simulink model "Mechanical_part_only"  (Simulink 7.5)
settings: Solver=ode4  StartTime=0.0  StopTime=10.0  FixedStep=0.05  RelTol=1e-3
settings Model: Creator=Slim  LastModifiedBy=Slim

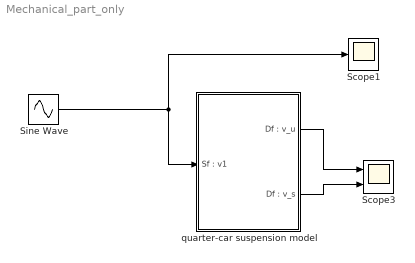
== system Mechanical_part_only ==
  Scope1 : Scope
      settings: YMin=6.25e-037  YMax=8.75e-037
  Scope3 : Scope  NumInputPorts=2
      settings: YMin=-5~-5  YMax=5~5
  Sine Wave : Sin  Amplitude=0.08*pi  Bias=0  Frequency=2*pi  Phase=pi/2  Samples=10  SampleTime=0  Offset=0
  quarter-car suspension model : Subsystem
  wires:
  Sine Wave/1 -> Scope1/1, quarter-car suspension model/1("Sf : v1")
  quarter-car suspension model/1("Df : v_u") -> Scope3/1
  quarter-car suspension model/2("Df : v_s") -> Scope3/2

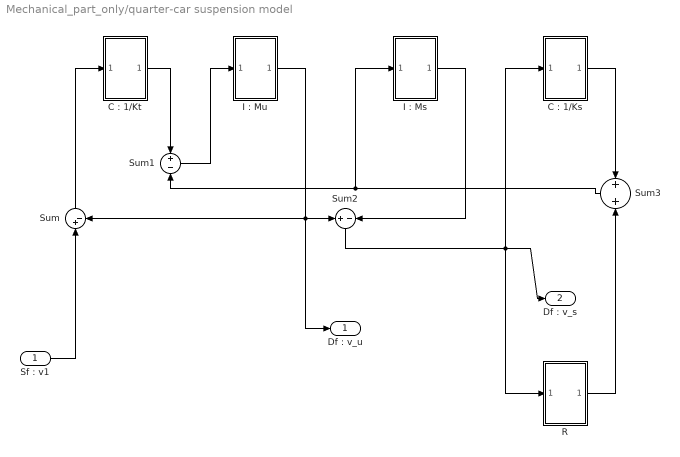
== system Mechanical_part_only/quarter-car suspension model ==
  "Sf : v1" : Inport  OutDataType=fixdt(1, 16)  OutScaling=2^0
  "C : 1/Ks" : Subsystem
  "C : 1/Kt" : Subsystem
  "I : Ms" : Subsystem
  "I : Mu" : Subsystem
  R : Subsystem
  Sum : Sum  Inputs=|+-  OutDataType=fixdt(1, 16)  OutScaling=2^0
  Sum1 : Sum  Inputs=+-  OutDataType=fixdt(1, 16)  OutScaling=2^0
  Sum2 : Sum  Inputs=+-  OutDataType=fixdt(1, 16)  OutScaling=2^0
  Sum3 : Sum  OutDataType=fixdt(1, 16)  OutScaling=2^0
  "Df : v_u" : Outport  OutDataType=fixdt(1, 16)  OutScaling=2^0
  "Df : v_s" : Outport  Port=2  OutDataType=fixdt(1, 16)  OutScaling=2^0
  wires:
  R/1(e23) -> Sum3/2
  "C : 1/Ks"/1(e21) -> Sum3/1
  Sum2/1 -> "Df : v_s"/1, R/1(f23), "C : 1/Ks"/1(f21)
  Sum3/1 -> "I : Ms"/1(e24), Sum1/2
  "I : Ms"/1(f24) -> Sum2/2
  "I : Mu"/1(f26) -> "Df : v_u"/1, Sum/2, Sum2/1
  Sum1/1 -> "I : Mu"/1(e26)
  "C : 1/Kt"/1(e28) -> Sum1/1
  Sum/1 -> "C : 1/Kt"/1(f28)
  "Sf : v1"/1 -> Sum/1

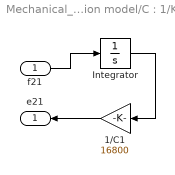
== system Mechanical_part_only/quarter-car suspension model/C : 1/Ks ==
  f21 : Inport  OutDataType=fixdt(1, 16)  OutScaling=2^0
  1/C1 : Gain  Gain=16800  ParameterDataType=fixdt(1, 16)  ParameterScaling=2^0  OutDataType=fixdt(1, 16)  OutScaling=2^0
  Integrator : Integrator
  e21 : Outport  OutDataType=fixdt(1, 16)  OutScaling=2^0
  wires:
  f21/1 -> Integrator/1
  Integrator/1 -> 1/C1/1
  1/C1/1 -> e21/1

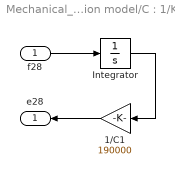
== system Mechanical_part_only/quarter-car suspension model/C : 1/Kt ==
  f28 : Inport  OutDataType=fixdt(1, 16)  OutScaling=2^0
  1/C1 : Gain  Gain=190000  ParameterDataType=fixdt(1, 16)  ParameterScaling=2^0  OutDataType=fixdt(1, 16)  OutScaling=2^0
  Integrator : Integrator
  e28 : Outport  OutDataType=fixdt(1, 16)  OutScaling=2^0
  wires:
  1/C1/1 -> e28/1
  Integrator/1 -> 1/C1/1
  f28/1 -> Integrator/1

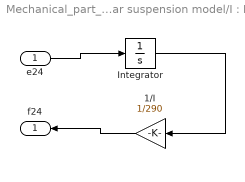
== system Mechanical_part_only/quarter-car suspension model/I : Ms ==
  e24 : Inport  OutDataType=fixdt(1, 16)  OutScaling=2^0
  1/I : Gain  Gain=1/290  ParameterDataType=fixdt(1, 16)  ParameterScaling=2^0  OutDataType=fixdt(1, 16)  OutScaling=2^0
  Integrator : Integrator
  f24 : Outport  OutDataType=fixdt(1, 16)  OutScaling=2^0
  wires:
  e24/1 -> Integrator/1
  Integrator/1 -> 1/I/1
  1/I/1 -> f24/1

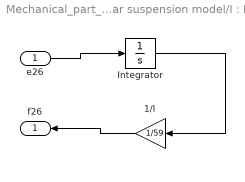
== system Mechanical_part_only/quarter-car suspension model/I : Mu ==
  e26 : Inport  OutDataType=fixdt(1, 16)  OutScaling=2^0
  1/I : Gain  Gain=1/59  ParameterDataType=fixdt(1, 16)  ParameterScaling=2^0  OutDataType=fixdt(1, 16)  OutScaling=2^0
  Integrator : Integrator
  f26 : Outport  OutDataType=fixdt(1, 16)  OutScaling=2^0
  wires:
  1/I/1 -> f26/1
  Integrator/1 -> 1/I/1
  e26/1 -> Integrator/1

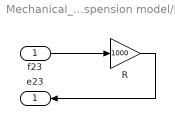
== system Mechanical_part_only/quarter-car suspension model/R ==
  f23 : Inport  OutDataType=fixdt(1, 16)  OutScaling=2^0
  R : Gain  Gain=1000  ParameterDataType=fixdt(1, 16)  ParameterScaling=2^0  OutDataType=fixdt(1, 16)  OutScaling=2^0
  e23 : Outport  OutDataType=fixdt(1, 16)  OutScaling=2^0
  wires:
  f23/1 -> R/1
  R/1 -> e23/1
